simulink model "Pract5_2"  (Simulink 7.2)
settings: Solver=ode45  StartTime=0.0  StopTime=0.001  RelTol=1e-3
libraries: commrandsrc2 x1
settings Model: Creator=Labcom  LastModifiedBy=Labcom

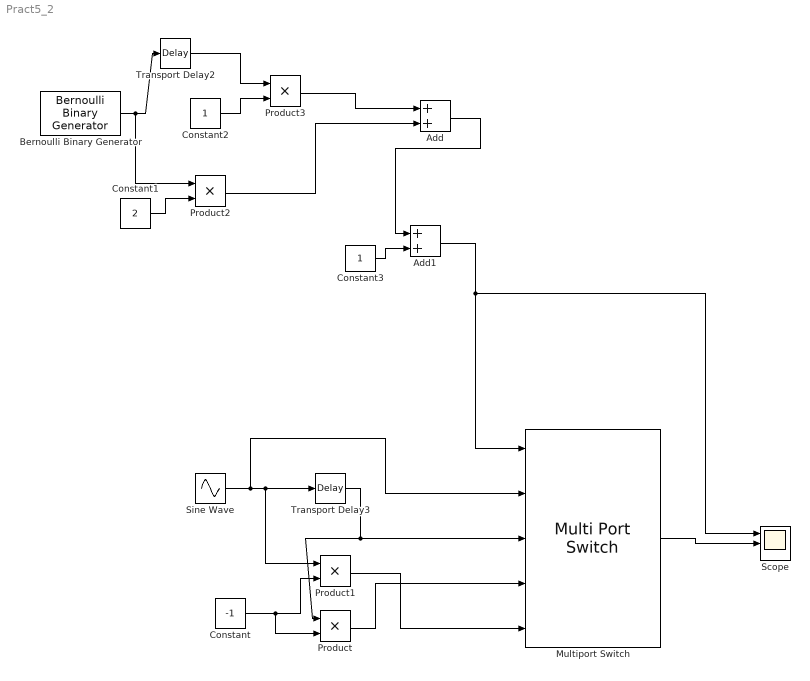
== system Pract5_2 ==
  Add : Sum  OutDataType=sfix(16)  OutScaling=2^-10
  Add1 : Sum  OutDataType=sfix(16)  OutScaling=2^-10
  Bernoulli Binary Generator : commrandsrc2/Bernoulli Binary Generator  DialogController=commDDGCreate  DialogControllerArgs=DataTag0  SystemSampleTime=-1  P=0.5  seed=35  Ts=0.00001  frameBased=off  sampPerFrame=1  orient=off  outDataType=double
  Constant : Constant  Value=-1  OutDataType=sfix(16)  OutScaling=2^0
  Constant1 : Constant  Value=2  OutDataType=sfix(16)  OutScaling=2^0
  Constant2 : Constant  OutDataType=sfix(16)  OutScaling=2^0
  Constant3 : Constant  OutDataType=sfix(16)  OutScaling=2^0
  Multiport Switch : MultiPortSwitch  Inputs=4  OutDataType=sfix(16)  OutScaling=2^0
  Product{,1..3} (4 alike) : Product  OutDataType=sfix(16)  OutScaling=2^0  RndMeth=Zero
  Scope : Scope  NumInputPorts=3
      settings: YMin=-5~-5~-5  YMax=5~5~5  MaxDataPoints=100000
  Sine Wave : Sin  Frequency=2*pi*1000000  SampleTime=0.00000001
  Transport Delay2 : TransportDelay  DelayTime=0.00001
  Transport Delay3 : TransportDelay  DelayTime=0.000001/4
  wires:
  Sine Wave/1 -> Transport Delay3/1, Product1/1, Multiport Switch/2
  Transport Delay3/1 -> Product/1, Multiport Switch/3
  Constant/1 -> Product1/2, Product/2
  Bernoulli Binary Generator/1 -> Transport Delay2/1, Product2/1
  Product1/1 -> Multiport Switch/5
  Product/1 -> Multiport Switch/4
  Transport Delay2/1 -> Product3/1
  Constant1/1 -> Product2/2
  Constant2/1 -> Product3/2
  Product3/1 -> Add/1
  Product2/1 -> Add/2
  Add/1 -> Add1/1
  Constant3/1 -> Add1/2
  Add1/1 -> Multiport Switch/1, Scope/1
  Multiport Switch/1 -> Scope/2
